simulink model "tolgaotonomyeni"  (R2022a)
settings: Solver=VariableStepAuto  StartTime=0.0  StopTime=100  RelTol=1e-3
values from neighbouring files (symbols this model uses):
  L = 3    [tolgaotonom.m]
  ld = 4    [tolgaotonom.m]
  psi_o = 0    [tolgaotonom.m]
  s = size(xRef)    [tolgaotonom.m]
  vel = lookUpt(2:27,2:32)    [tolgaotonom.m]
  X_o = refPose(1,1)    [tolgaotonom.m]
  xlt = lookUpt(2:27,1)    [tolgaotonom.m]
  xRef = refPose(:,1)    [tolgaotonom.m]
  Y_o = -refPose(1,2)    [tolgaotonom.m]
  ylt = lookUpt(1,2:32)    [tolgaotonom.m]
  yRef = -refPose(:,2)    [tolgaotonom.m]
libraries: autolibutils x4, autolibshared x3, vehdynlibviscommon x1, robotalgslib x1, simulink x1, sim3dlib x1, vdynlib x1
(part 3 of 3)

== system tolgaotonomyeni/Powertrain & Driveline/Driveline/RWD ==
  TPowertrain : Inport
  RWD : Gain  Gain=[0;0;1;1]
  TAxles : Outport  VectorParamsAs1DForOutWhenUnconnected=off
  wires:
  TPowertrain/1 -> RWD/1
  RWD/1 -> TAxles/1
